simulink library "lib_SignalDiagnostic"  (R2017a)
settings: Solver=VariableStepAuto  StartTime=0.0  StopTime=10.0  RelTol=1e-3
libraries: simulink x35
settings Model: Creator=Di Russo  LastModifiedBy=Di Russo

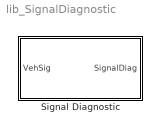
== system lib_SignalDiagnostic ==
  Signal Diagnostic : Subsystem

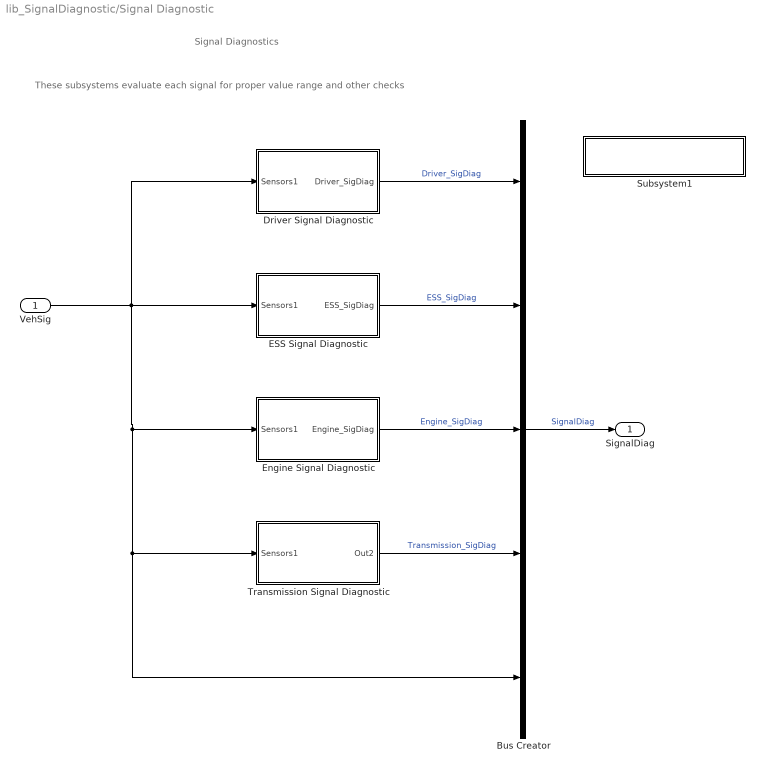
== system lib_SignalDiagnostic/Signal Diagnostic ==
  note: These subsystems evaluate each signal for proper value range and other checks
  note: Signal Diagnostics
  VehSig : Inport
  Bus Creator : BusCreator  Inputs=5
  Driver Signal Diagnostic : Subsystem
  ESS Signal Diagnostic : Subsystem
  Engine Signal Diagnostic : Subsystem
  Subsystem1 : Subsystem
      mask Display: fprintf('Signal Naming Rule')
  Transmission Signal Diagnostic : Subsystem
  SignalDiag : Outport
  wires:
  VehSig/1 -> ESS Signal Diagnostic/1(Sensors1), Driver Signal Diagnostic/1(Sensors1), Engine Signal Diagnostic/1(Sensors1), Bus Creator/5, Transmission Signal Diagnostic/1(Sensors1)
  Driver Signal Diagnostic/1(Driver_SigDiag) -> Bus Creator/1  "Driver_SigDiag"
  ESS Signal Diagnostic/1(ESS_SigDiag) -> Bus Creator/2  "ESS_SigDiag"
  Engine Signal Diagnostic/1(Engine_SigDiag) -> Bus Creator/3  "Engine_SigDiag"
  Transmission Signal Diagnostic/1(Out2) -> Bus Creator/4  "Transmission_SigDiag"
  Bus Creator/1 -> SignalDiag/1  "SignalDiag"

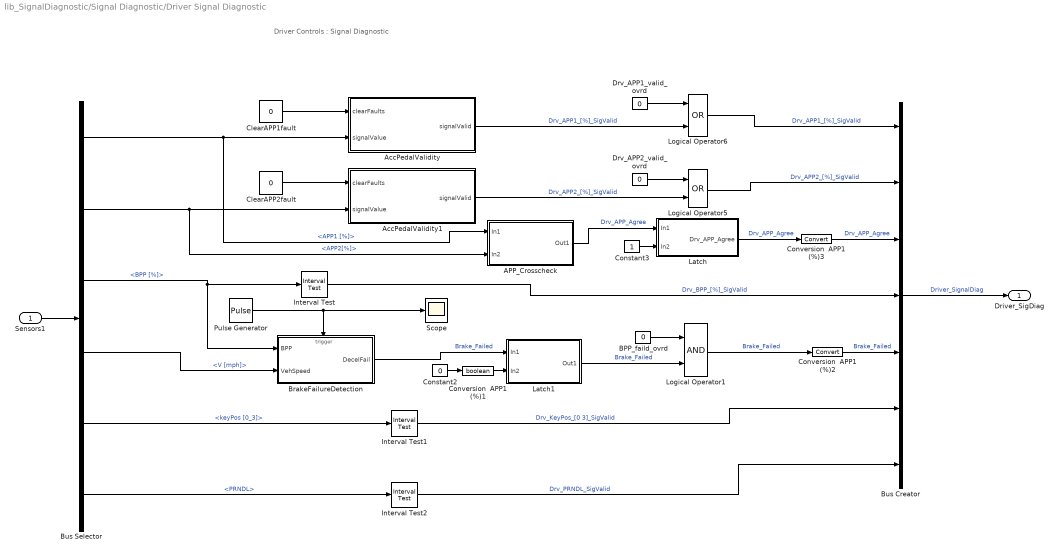
== system lib_SignalDiagnostic/Signal Diagnostic/Driver Signal Diagnostic ==
  note: Driver Controls : Signal Diagnostic
  Sensors1 : Inport
  APP_Crosscheck : Subsystem
  AccPedalValidity : Stateflow chart  TreatAsAtomicUnit=on
  AccPedalValidity1 : Stateflow chart  TreatAsAtomicUnit=on
  BPP_faild_ovrd : Constant  Value=0  OutDataTypeStr=boolean
  BrakeFailureDetection : Subsystem
  Bus Creator : BusCreator  Inputs=7
  Bus Selector : BusSelector  OutputSignals=DriverControls_Conv.APP1 [%],DriverControls_Conv.APP2[%],DriverControls_Conv.BPP [%],DriverControls_Conv.V [mph],DriverControls_Conv.keyPos [0_3],DriverControls_Conv.PRNDL
  ClearAPP1fault : Constant  Value=0
  ClearAPP2fault : Constant  Value=0
  Constant2 : Constant  Value=0
  Constant3 : Constant  OutDataTypeStr=boolean
  Conversion  APP1 (%)1 : DataTypeConversion  OutDataTypeStr=boolean
  Conversion  APP1 (%)2 : DataTypeConversion
  Conversion  APP1 (%)3 : DataTypeConversion
  Drv_APP1_valid_ovrd : Constant  Value=0  OutDataTypeStr=boolean
  Drv_APP2_valid_ovrd : Constant  Value=0  OutDataTypeStr=boolean
  Interval Test : simulink/Logic and Bit Operations/Interval Test  IntervalClosedRight=on  uplimit=100  IntervalClosedLeft=on  lowlimit=0  OutDataTypeStr=boolean
  Interval Test1 : simulink/Logic and Bit Operations/Interval Test  IntervalClosedRight=on  uplimit=3  IntervalClosedLeft=on  lowlimit=0  OutDataTypeStr=boolean
  Interval Test2 : simulink/Logic and Bit Operations/Interval Test  IntervalClosedRight=on  uplimit=4  IntervalClosedLeft=on  lowlimit=0  OutDataTypeStr=boolean
  Latch : Subsystem
  Latch1 : Subsystem
  Logical Operator1 : Logic  AllPortsSameDT=off  OutDataTypeStr=boolean
  Logical Operator5 : Logic  Operator=OR  AllPortsSameDT=off  OutDataTypeStr=boolean
  Logical Operator6 : Logic  Operator=OR  AllPortsSameDT=off  OutDataTypeStr=boolean
  Pulse Generator : DiscretePulseGenerator  PulseType=Time based  Period=0.1  PulseWidth=10
  Scope : Scope
  Driver_SigDiag : Outport
  wires:
  Sensors1/1 -> Bus Selector/1
  Bus Selector/1 -> AccPedalValidity/2(signalValue), APP_Crosscheck/1(In1)  "<APP1 [%]>"
  Bus Selector/2 -> AccPedalValidity1/2(signalValue), APP_Crosscheck/2(In2)  "<APP2[%]>"
  ClearAPP1fault/1 -> AccPedalValidity/1(clearFaults)
  ClearAPP2fault/1 -> AccPedalValidity1/1(clearFaults)
  Bus Selector/3 -> Interval Test/1, BrakeFailureDetection/1(BPP)  "<BPP [%]>"
  Bus Selector/5 -> Interval Test1/1  "<keyPos [0_3]>"
  Logical Operator6/1 -> Bus Creator/1  "Drv_APP1_[%]_SigValid"
  Interval Test/1 -> Bus Creator/4  "Drv_BPP_[%]_SigValid"
  Logical Operator5/1 -> Bus Creator/2  "Drv_APP2_[%]_SigValid"
  Bus Creator/1 -> Driver_SigDiag/1  "Driver_SignalDiag"
  Bus Selector/6 -> Interval Test2/1  "<PRNDL>"
  Constant3/1 -> Latch/2(In2)
  APP_Crosscheck/1(Out1) -> Latch/1(In1)  "Drv_APP_Agree"
  Bus Selector/4 -> BrakeFailureDetection/2(VehSpeed)  "<V [mph]>"
  Constant2/1 -> Conversion  APP1 (%)1/1
  Conversion  APP1 (%)1/1 -> Latch1/2(In2)
  BrakeFailureDetection/1(DecelFail) -> Latch1/1(In1)  "Brake_Failed"
  Interval Test2/1 -> Bus Creator/7  "Drv_PRNDL_SigValid"
  Drv_APP2_valid_ovrd/1 -> Logical Operator5/1
  AccPedalValidity1/1(signalValid) -> Logical Operator5/2  "Drv_APP2_[%]_SigValid"
  Drv_APP1_valid_ovrd/1 -> Logical Operator6/1
  AccPedalValidity/1(signalValid) -> Logical Operator6/2  "Drv_APP1_[%]_SigValid"
  Conversion  APP1 (%)3/1 -> Bus Creator/3  "Drv_APP_Agree"
  Conversion  APP1 (%)2/1 -> Bus Creator/5  "Brake_Failed"
  Interval Test1/1 -> Bus Creator/6  "Drv_KeyPos_[0 3]_SigValid"
  Latch/1(Drv_APP_Agree) -> Conversion  APP1 (%)3/1  "Drv_APP_Agree"
  Logical Operator1/1 -> Conversion  APP1 (%)2/1  "Brake_Failed"
  Latch1/1(Out1) -> Logical Operator1/2  "Brake_Failed"
  BPP_faild_ovrd/1 -> Logical Operator1/1
  Pulse Generator/1 -> BrakeFailureDetection/Trigger, Scope/1

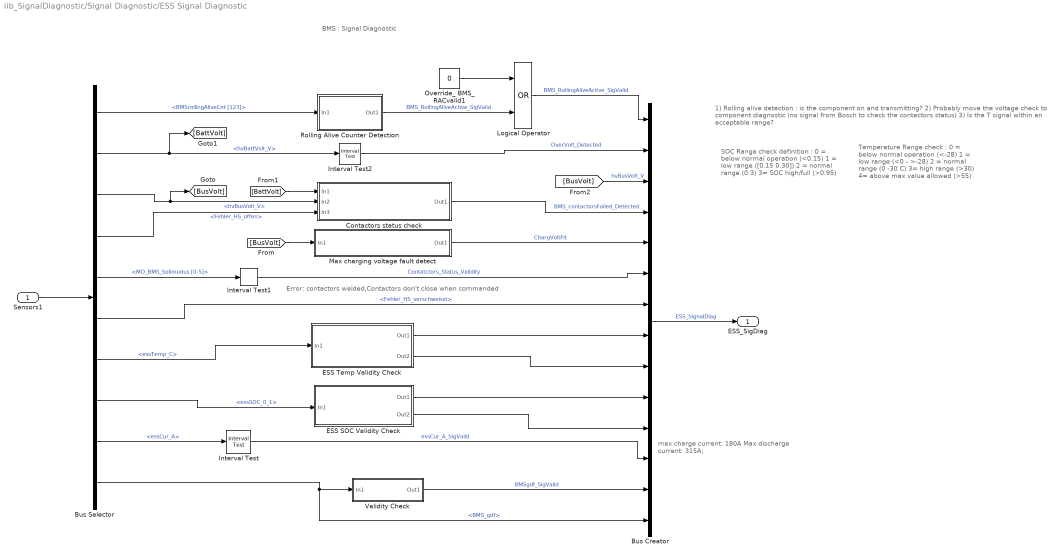
== system lib_SignalDiagnostic/Signal Diagnostic/ESS Signal Diagnostic ==
  note: max charge current: 180A
      | Max discharge current: 315A;
  note: Error: contactors welded,Contactors don't close when commanded
  note: Temperature Range check :
      | 0 = below normal operation (<-28)
      | 1 = low range (<0 - >-28)
      | 2 = normal range (0 -30 C)
      | 3= high range (>30)
      | 4= above max value allowed (>55)
  note: SOC Range check definition :
      | 0 = below normal operation (<0.15)
      | 1 = low range ([0.15 0.30])
      | 2 = normal range (0.3)
      | 3= SOC high/full (>0.95)
  note: 1) Rolling alive detection : is the component on and transmitting?
      | 2) Probably move the voltage check to component diagnostic (no signal from Bosch to check the contactors status)
      | 3) Is  the T signal within an acceptable range?
  note: BMS : Signal Diagnostic
  Sensors1 : Inport
  Bus Creator : BusCreator  Inputs=14
  Bus Selector : BusSelector  OutputSignals=BMS_Conv.BMSrollingAliveCnt [123],BMS_Conv.hvBattVolt_V,BMS_Conv.hvBusVolt_V,BMS_Conv.Fehler_HS_offen,BMS_Conv.MO_BMS_Sollmodus [0-5],BMS_Conv.Fehler_HS_verschweisst,BMS_Conv.essTemp_C,BMS_Conv.essSOC_0_1,BMS_Conv.essCur_A,BMS_Conv.BMS_gdf
  Contactors status check : Subsystem
  ESS SOC Validity Check : Subsystem
  ESS Temp Validity Check : Subsystem
  Interval Test : simulink/Logic and Bit Operations/Interval Test  IntervalClosedRight=on  uplimit=180  IntervalClosedLeft=on  lowlimit=-315  OutDataTypeStr=boolean
  Interval Test1 : simulink/Logic and Bit Operations/Interval Test  IntervalClosedRight=on  uplimit=7  IntervalClosedLeft=on  lowlimit=0  OutDataTypeStr=boolean
  Interval Test2 : simulink/Logic and Bit Operations/Interval Test  IntervalClosedRight=on  uplimit=430  IntervalClosedLeft=on  lowlimit=291  OutDataTypeStr=boolean
  Logical Operator : Logic  Operator=OR  AllPortsSameDT=off  OutDataTypeStr=boolean
  Max charging voltage fault detect : Subsystem
  Override_ BMS_RACvalid1 : Constant  Value=0
  Rolling Alive Counter Detection : Subsystem
  Validity Check : Subsystem
  ESS_SigDiag : Outport
  wires:
  Sensors1/1 -> Bus Selector/1
  Bus Selector/1 -> Rolling Alive Counter Detection/1(In1)  "<BMSrollingAliveCnt [123]>"
  Logical Operator/1 -> Bus Creator/1  "BMS_RollingAliveActive_SigValid"
  Bus Selector/2 -> Interval Test2/1, [BattVolt]  "<hvBattVolt_V>"
  Bus Creator/1 -> ESS_SigDiag/1  "ESS_SignalDiag"
  Bus Selector/9 -> Interval Test/1  "<essCur_A>"
  Interval Test/1 -> Bus Creator/12  "essCur_A_SigValid"
  Bus Selector/10 -> Bus Creator/14, Validity Check/1(In1)  "<BMS_gdf>"
  Validity Check/1(Out1) -> Bus Creator/13  "BMSgdf_SigValid"
  Bus Selector/8 -> ESS SOC Validity Check/1(In1)  "<essSOC_0_1>"
  ESS SOC Validity Check/1(Out1) -> Bus Creator/10
  ESS SOC Validity Check/2(Out2) -> Bus Creator/11
  Bus Selector/7 -> ESS Temp Validity Check/1(In1)  "<essTemp_C>"
  ESS Temp Validity Check/1(Out1) -> Bus Creator/8
  ESS Temp Validity Check/2(Out2) -> Bus Creator/9
  Bus Selector/3 -> Contactors status check/2(In2), [BusVolt]  "<hvBusVolt_V>"
  Bus Selector/4 -> Contactors status check/3(In3)  "<Fehler_HS_offen>"
  Contactors status check/1(Out1) -> Bus Creator/4  "BMS_contactorsFailed_Detected"
  Bus Selector/6 -> Bus Creator/7  "<Fehler_HS_verschweisst>"
  Bus Selector/5 -> Interval Test1/1  "<MO_BMS_Sollmodus [0-5]>"
  Interval Test1/1 -> Bus Creator/6  "Contatctors_Status_Validity"
  Interval Test2/1 -> Bus Creator/2  "OverVolt_Detected"
  [BattVolt] -> Contactors status check/1(In1)
  [BusVolt] -> Max charging voltage fault detect/1(In1)
  Max charging voltage fault detect/1(Out1) -> Bus Creator/5  "ChargVoltFlt"
  [BusVolt] -> Bus Creator/3  "hvBusVolt_V"
  Rolling Alive Counter Detection/1(Out1) -> Logical Operator/2  "BMS_RollingAliveActive_SigValid"
  Override_ BMS_RACvalid1/1 -> Logical Operator/1

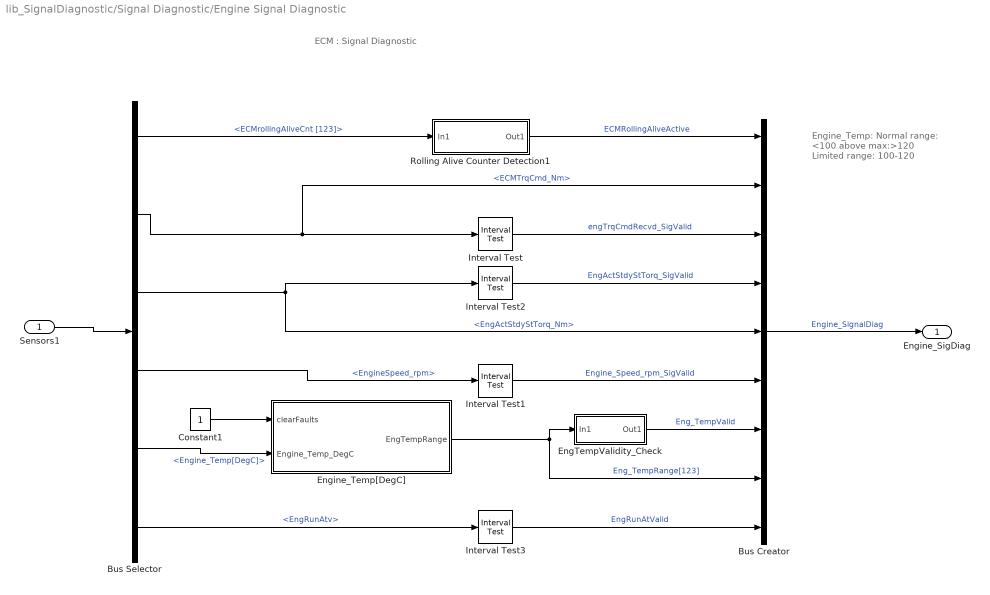
== system lib_SignalDiagnostic/Signal Diagnostic/Engine Signal Diagnostic ==
  note: ECM : Signal Diagnostic
  note: Engine_Temp:
      | Normal range: <100
      | above max:>120
      | Limited range: 100-120
  Sensors1 : Inport
  Bus Creator : BusCreator  Inputs=9
  Bus Selector : BusSelector  OutputSignals=ECM_Conv.ECMrollingAliveCnt [123],ECM_Conv.ECMTrqCmd_Nm,ECM_Conv.EngActStdyStTorq_Nm,ECM_Conv.EngineSpeed_rpm,ECM_Conv.Engine_Temp[DegC],ECM_Conv.EngRunAtv
  Constant1 : Constant
  EngTempValidity_Check : Subsystem
  Engine_Temp[DegC] : Stateflow chart  TreatAsAtomicUnit=on
  Interval Test : simulink/Logic and Bit Operations/Interval Test  IntervalClosedRight=on  uplimit=233  IntervalClosedLeft=on  lowlimit=0  OutDataTypeStr=boolean
  Interval Test1 : simulink/Logic and Bit Operations/Interval Test  IntervalClosedRight=on  uplimit=6500  IntervalClosedLeft=on  lowlimit=0  OutDataTypeStr=boolean
  Interval Test2 : simulink/Logic and Bit Operations/Interval Test  IntervalClosedRight=on  uplimit=233  IntervalClosedLeft=on  lowlimit=0  OutDataTypeStr=boolean
  Interval Test3 : simulink/Logic and Bit Operations/Interval Test  IntervalClosedRight=on  uplimit=1  IntervalClosedLeft=on  lowlimit=0  OutDataTypeStr=boolean
  Rolling Alive Counter Detection1 : Subsystem
  Engine_SigDiag : Outport
  wires:
  Sensors1/1 -> Bus Selector/1
  Bus Selector/1 -> Rolling Alive Counter Detection1/1(In1)  "<ECMrollingAliveCnt [123]>"
  Rolling Alive Counter Detection1/1(Out1) -> Bus Creator/1  "ECMRollingAliveActive"
  Bus Selector/2 -> Bus Creator/2, Interval Test/1  "<ECMTrqCmd_Nm>"
  Interval Test/1 -> Bus Creator/3  "engTrqCmdRecvd_SigValid"
  Bus Creator/1 -> Engine_SigDiag/1  "Engine_SignalDiag"
  Bus Selector/4 -> Interval Test1/1  "<EngineSpeed_rpm>"
  Interval Test1/1 -> Bus Creator/6  "Engine_Speed_rpm_SigValid"
  Bus Selector/3 -> Bus Creator/5, Interval Test2/1  "<EngActStdyStTorq_Nm>"
  Interval Test2/1 -> Bus Creator/4  "EngActStdyStTorq_SigValid"
  Bus Selector/5 -> Engine_Temp[DegC]/2(Engine_Temp_DegC)  "<Engine_Temp[DegC]>"
  Bus Selector/6 -> Interval Test3/1  "<EngRunAtv>"
  Interval Test3/1 -> Bus Creator/9  "EngRunAtValid"
  Constant1/1 -> Engine_Temp[DegC]/1(clearFaults)
  Engine_Temp[DegC]/1(EngTempRange) -> EngTempValidity_Check/1(In1), Bus Creator/8  "Eng_TempRange[123]"
  EngTempValidity_Check/1(Out1) -> Bus Creator/7  "Eng_TempValid"

== system lib_SignalDiagnostic/Signal Diagnostic/Subsystem1 ==
  note: Signal Valid Setting Rule
      | xxx_yyy_[z]_SigValid could be 0 or 1
      | 0: signal invalid
      | 1: signal vaild
  note: Signal Naming Rule
      | Example: xxx_yyy_[z]_SigValid
      | xxx: source of the signal (Drv, Clu, BCM, ECM, TCM, BMS and MCU)
      | yyy: description of the signal
      | z: unit of the signal (V, A, Nm, m/s, %, 01, 0123, etc.)

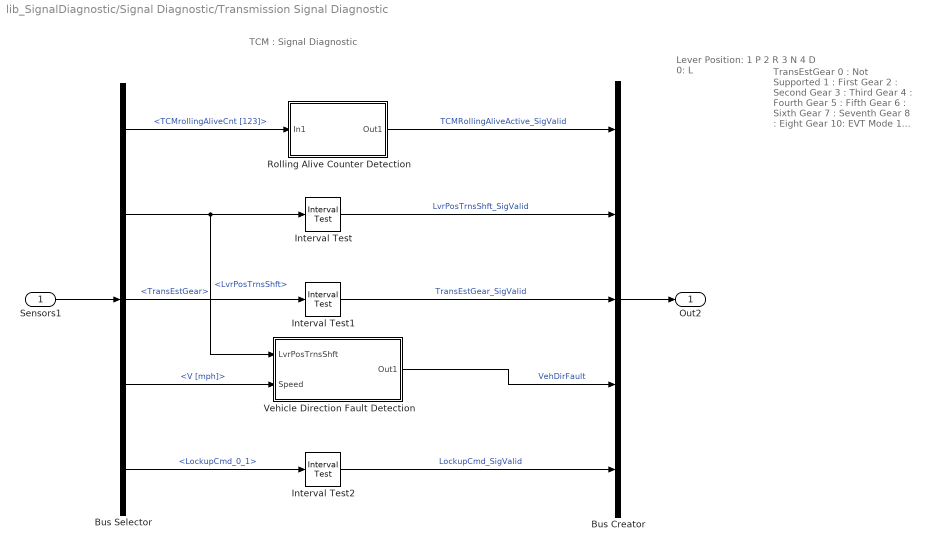
== system lib_SignalDiagnostic/Signal Diagnostic/Transmission Signal Diagnostic ==
  note: TCM : Signal Diagnostic
  note: TransEstGear
      | 0 : Not Supported
      | 1 : First Gear
      | 2 : Second Gear
      | 3 : Third Gear
      | 4 : Fourth Gear
      | 5 : Fifth Gear
      | 6 : Sixth Gear
      | 7 : Seventh Gear
      | 8 : Eight Gear
      | 10: EVT Mode 1
      | 11: EVT Mode 2
      | 12: CVT Forward Gear
      | 13: Neutral Gear
      | 14: Reverse Gear
      | 15: Park Gear
  note: Lever Position:
      | 1 P
      | 2 R
      | 3 N
      | 4 D
      | 0: L
  Sensors1 : Inport
  Bus Creator : BusCreator  Inputs=5
  Bus Selector : BusSelector  OutputSignals=TCM_Conv.TCMrollingAliveCnt [123],TCM_Conv.LvrPosTrnsShft,TCM_Conv.TransEstGear,DriverControls_Conv.V [mph],TCM_Conv.LockupCmd_0_1
  Interval Test : simulink/Logic and Bit Operations/Interval Test  IntervalClosedRight=on  uplimit=4  IntervalClosedLeft=on  lowlimit=0  OutDataTypeStr=boolean
  Interval Test1 : simulink/Logic and Bit Operations/Interval Test  IntervalClosedRight=on  uplimit=15  IntervalClosedLeft=on  lowlimit=0  OutDataTypeStr=boolean
  Interval Test2 : simulink/Logic and Bit Operations/Interval Test  IntervalClosedRight=on  uplimit=1  IntervalClosedLeft=on  lowlimit=0  OutDataTypeStr=boolean
  Rolling Alive Counter Detection : Subsystem
  Vehicle Direction Fault Detection : Subsystem
  Out2 : Outport
  wires:
  Bus Selector/4 -> Vehicle Direction Fault Detection/2(Speed)  "<V [mph]>"
  Sensors1/1 -> Bus Selector/1
  Bus Selector/1 -> Rolling Alive Counter Detection/1(In1)  "<TCMrollingAliveCnt [123]>"
  Rolling Alive Counter Detection/1(Out1) -> Bus Creator/1  "TCMRollingAliveActive_SigValid"
  Bus Creator/1 -> Out2/1
  Bus Selector/2 -> Vehicle Direction Fault Detection/1(LvrPosTrnsShft), Interval Test/1  "<LvrPosTrnsShft>"
  Bus Selector/3 -> Interval Test1/1  "<TransEstGear>"
  Bus Selector/5 -> Interval Test2/1  "<LockupCmd_0_1>"
  Interval Test/1 -> Bus Creator/2  "LvrPosTrnsShft_SigValid"
  Interval Test1/1 -> Bus Creator/3  "TransEstGear_SigValid"
  Interval Test2/1 -> Bus Creator/5  "LockupCmd_SigValid"
  Vehicle Direction Fault Detection/1(Out1) -> Bus Creator/4  "VehDirFault"

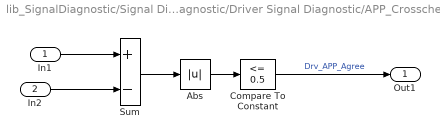
== system lib_SignalDiagnostic/Signal Diagnostic/Driver Signal Diagnostic/APP_Crosscheck ==
  In1 : Inport
  In2 : Inport  Port=2
  Abs : Abs
  Compare To Constant : simulink/Logic and Bit Operations/Compare To Constant  relop=<=  const=0.5  OutDataTypeStr=boolean
  Sum : Sum  Inputs=+-
  Out1 : Outport
  wires:
  Sum/1 -> Abs/1
  Abs/1 -> Compare To Constant/1
  In1/1 -> Sum/1
  In2/1 -> Sum/2
  Compare To Constant/1 -> Out1/1  "Drv_APP_Agree"

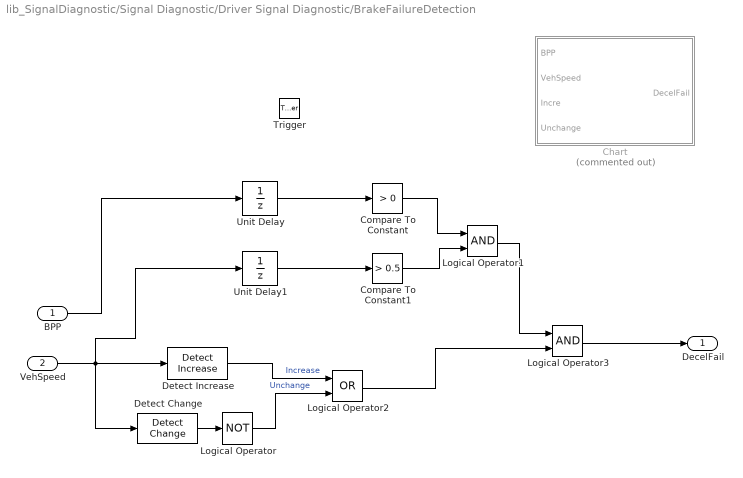
== system lib_SignalDiagnostic/Signal Diagnostic/Driver Signal Diagnostic/BrakeFailureDetection ==
  BPP : Inport
  VehSpeed : Inport  Port=2
  Trigger : TriggerPort  VariantControl=Variant  PortDimensions=1
  Chart : Stateflow chart  Commented=on  TreatAsAtomicUnit=on
  Compare To Constant : simulink/Logic and Bit Operations/Compare To Constant  relop=>  const=0  OutDataTypeStr=boolean
  Compare To Constant1 : simulink/Logic and Bit Operations/Compare To Constant  relop=>  const=0.5  OutDataTypeStr=boolean
  Detect Change : simulink/Logic and Bit Operations/Detect Change  vinit=0  InputProcessing=Inherited  OutDataTypeStr=boolean
  Detect Increase : simulink/Logic and Bit Operations/Detect Increase  vinit=0.0  InputProcessing=Inherited  OutDataTypeStr=boolean
  Logical Operator : Logic  Operator=NOT  AllPortsSameDT=off  OutDataTypeStr=boolean
  Logical Operator1 : Logic  AllPortsSameDT=off  OutDataTypeStr=boolean
  Logical Operator2 : Logic  Operator=OR  AllPortsSameDT=off  OutDataTypeStr=boolean
  Logical Operator3 : Logic  AllPortsSameDT=off  OutDataTypeStr=boolean
  Unit Delay : UnitDelay  SampleTime=-1
  Unit Delay1 : UnitDelay  SampleTime=-1
  DecelFail : Outport
  wires:
  VehSpeed/1 -> Unit Delay1/1, Detect Change/1, Detect Increase/1
  Detect Change/1 -> Logical Operator/1
  Compare To Constant/1 -> Logical Operator1/1
  Compare To Constant1/1 -> Logical Operator1/2
  BPP/1 -> Unit Delay/1
  Logical Operator1/1 -> Logical Operator3/1
  Detect Increase/1 -> Logical Operator2/1  "Increase"
  Logical Operator/1 -> Logical Operator2/2  "Unchange"
  Unit Delay/1 -> Compare To Constant/1
  Unit Delay1/1 -> Compare To Constant1/1
  Logical Operator2/1 -> Logical Operator3/2
  Logical Operator3/1 -> DecelFail/1

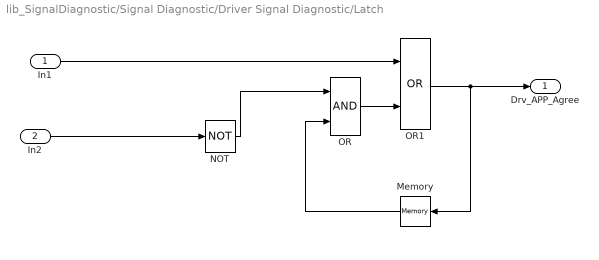
== system lib_SignalDiagnostic/Signal Diagnostic/Driver Signal Diagnostic/Latch ==
  In1 : Inport
  In2 : Inport  Port=2
  Memory : Memory
  NOT : Logic  Operator=NOT  OutDataTypeStr=boolean
  OR : Logic  OutDataTypeStr=boolean
  OR1 : Logic  Operator=OR  OutDataTypeStr=boolean
  Drv_APP_Agree : Outport
  wires:
  In1/1 -> OR1/1
  OR/1 -> OR1/2
  OR1/1 -> Drv_APP_Agree/1, Memory/1
  NOT/1 -> OR/1
  Memory/1 -> OR/2
  In2/1 -> NOT/1

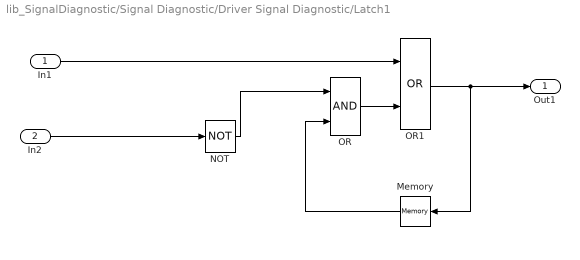
== system lib_SignalDiagnostic/Signal Diagnostic/Driver Signal Diagnostic/Latch1 ==
  In1 : Inport
  In2 : Inport  Port=2
  Memory : Memory
  NOT : Logic  Operator=NOT  OutDataTypeStr=boolean
  OR : Logic  OutDataTypeStr=boolean
  OR1 : Logic  Operator=OR  OutDataTypeStr=boolean
  Out1 : Outport
  wires:
  In2/1 -> NOT/1
  Memory/1 -> OR/2
  NOT/1 -> OR/1
  OR1/1 -> Memory/1, Out1/1
  OR/1 -> OR1/2
  In1/1 -> OR1/1

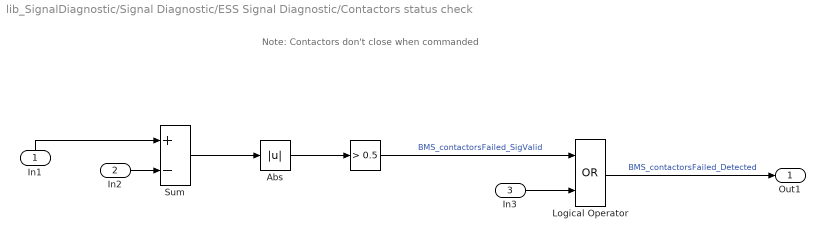
== system lib_SignalDiagnostic/Signal Diagnostic/ESS Signal Diagnostic/Contactors status check ==
  note: Note: Contactors don't close when commanded
  In1 : Inport
  In2 : Inport  Port=2
  In3 : Inport  Port=3
  " " : simulink/Logic and Bit Operations/Compare To Constant  relop=>  const=0.5  OutDataTypeStr=boolean
  Abs : Abs
  Logical Operator : Logic  Operator=OR  AllPortsSameDT=off  OutDataTypeStr=boolean
  Sum : Sum  Inputs=+-
  Out1 : Outport
  wires:
  " "/1 -> Logical Operator/1  "BMS_contactorsFailed_SigValid"
  In3/1 -> Logical Operator/2
  In2/1 -> Sum/2
  Abs/1 -> " "/1
  Sum/1 -> Abs/1
  Logical Operator/1 -> Out1/1  "BMS_contactorsFailed_Detected"
  In1/1 -> Sum/1

== system lib_SignalDiagnostic/Signal Diagnostic/ESS Signal Diagnostic/ESS SOC Validity Check ==
  In1 : Inport
  Constant1 : Constant
  essSOCValidity_Check : Subsystem
  essSOC_0_1Range : Stateflow chart  TreatAsAtomicUnit=on
  Out1 : Outport
  Out2 : Outport  Port=2
  wires:
  essSOCValidity_Check/1(Out1) -> Out1/1  "BMS_essSOC_0_1_SigValid"
  In1/1 -> essSOC_0_1Range/2(signalValue)
  Constant1/1 -> essSOC_0_1Range/1(clearFaults)
  essSOC_0_1Range/1(essSOCRange) -> Out2/1, essSOCValidity_Check/1(In1)

== system lib_SignalDiagnostic/Signal Diagnostic/ESS Signal Diagnostic/ESS Temp Validity Check ==
  In1 : Inport
  Constant : Constant
  essTsignalRange : Stateflow chart  TreatAsAtomicUnit=on
  essTsignalValidity_Check : Subsystem
  Out1 : Outport
  Out2 : Outport  Port=2
  wires:
  Constant/1 -> essTsignalRange/1(clearFaults)
  essTsignalValidity_Check/1(Out1) -> Out1/1  "BMS_essTemp_[degC]_SigValid"
  essTsignalRange/1(essTempRange) -> Out2/1, essTsignalValidity_Check/1(In1)  "essTempRange[0_4]"
  In1/1 -> essTsignalRange/2(signalValue)

== system lib_SignalDiagnostic/Signal Diagnostic/ESS Signal Diagnostic/Max charging voltage fault detect ==
  note: Note: When the ESS receives the energy from grid or regenerative braking,
      | the charging voltage to the inverter can not be bigger than 419V, otherwise the MCU will set to fault
  In1 : Inport
  " " : simulink/Logic and Bit Operations/Compare To Constant  relop=>  const=419  OutDataTypeStr=boolean
  Abs : Abs
  Compare To Zero : simulink/Logic and Bit Operations/Compare To Zero  relop=<  OutDataTypeStr=boolean
  Logical Operator : Logic  AllPortsSameDT=off  OutDataTypeStr=boolean
  Out1 : Outport
  wires:
  Compare To Zero/1 -> Logical Operator/2
  In1/1 -> Abs/1, Compare To Zero/1
  " "/1 -> Logical Operator/1
  Logical Operator/1 -> Out1/1
  Abs/1 -> " "/1

== system lib_SignalDiagnostic/Signal Diagnostic/ESS Signal Diagnostic/Rolling Alive Counter Detection ==
  In1 : Inport
  Chart : Stateflow chart  TreatAsAtomicUnit=on
  Constant : Constant  Value=0.01
  Constant1 : Constant  Value=0.01
  Detect Change : simulink/Logic and Bit Operations/Detect Change  vinit=1  InputProcessing=Inherited  OutDataTypeStr=boolean
  Out1 : Outport
  wires:
  Constant/1 -> Chart/2(CycleTime)
  Chart/1(flag) -> Out1/1
  Detect Change/1 -> Chart/1(PulseDetect)
  In1/1 -> Detect Change/1
  Constant1/1 -> Chart/3(tloop)

== system lib_SignalDiagnostic/Signal Diagnostic/ESS Signal Diagnostic/Validity Check ==
  In1 : Inport
  " Normal Operation" : simulink/Logic and Bit Operations/Compare To Constant  relop===  const=1  OutDataTypeStr=boolean
  Below Normal Operation : simulink/Logic and Bit Operations/Compare To Constant  relop===  const=0  OutDataTypeStr=boolean
  Logical Operator : Logic  Operator=OR  AllPortsSameDT=off  OutDataTypeStr=boolean
  Out1 : Outport
  wires:
  Logical Operator/1 -> Out1/1  "BMSgdf_SigValid"
  " Normal Operation"/1 -> Logical Operator/2
  Below Normal Operation/1 -> Logical Operator/1
  In1/1 -> " Normal Operation"/1, Below Normal Operation/1

== system lib_SignalDiagnostic/Signal Diagnostic/Engine Signal Diagnostic/EngTempValidity_Check ==
  In1 : Inport
  Above Normal Operation : simulink/Logic and Bit Operations/Compare To Constant  relop===  const=3  OutDataTypeStr=boolean
  Logical Operator1 : Logic  Operator=NOT  AllPortsSameDT=off  OutDataTypeStr=boolean
  Out1 : Outport
  wires:
  In1/1 -> Above Normal Operation/1
  Above Normal Operation/1 -> Logical Operator1/1
  Logical Operator1/1 -> Out1/1

== system lib_SignalDiagnostic/Signal Diagnostic/Engine Signal Diagnostic/Rolling Alive Counter Detection1 ==
  In1 : Inport
  Chart : Stateflow chart  TreatAsAtomicUnit=on
  Constant : Constant  Value=0.01
  Detect Change : simulink/Logic and Bit Operations/Detect Change  vinit=1  InputProcessing=Inherited  OutDataTypeStr=boolean
  Out1 : Outport
  wires:
  In1/1 -> Detect Change/1
  Detect Change/1 -> Chart/1(PulseDetect)
  Chart/1(flag) -> Out1/1
  Constant/1 -> Chart/2(CycleTime)

== system lib_SignalDiagnostic/Signal Diagnostic/Transmission Signal Diagnostic/Rolling Alive Counter Detection ==
  In1 : Inport
  Chart : Stateflow chart  TreatAsAtomicUnit=on
  Constant : Constant  Value=0.01
  Detect Change : simulink/Logic and Bit Operations/Detect Change  vinit=1  InputProcessing=Inherited  OutDataTypeStr=boolean
  Out1 : Outport
  wires:
  In1/1 -> Detect Change/1
  Detect Change/1 -> Chart/1(PulseDetect)
  Chart/1(flag) -> Out1/1
  Constant/1 -> Chart/2(CycleTime)

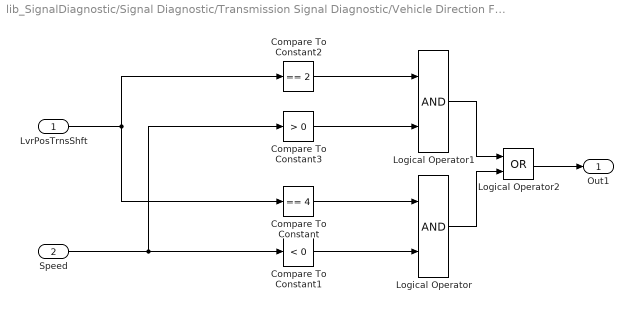
== system lib_SignalDiagnostic/Signal Diagnostic/Transmission Signal Diagnostic/Vehicle Direction Fault Detection ==
  LvrPosTrnsShft : Inport
  Speed : Inport  Port=2
  Compare To Constant : simulink/Logic and Bit Operations/Compare To Constant  relop===  const=4  OutDataTypeStr=boolean
  Compare To Constant1 : simulink/Logic and Bit Operations/Compare To Constant  relop=<  const=0  OutDataTypeStr=boolean
  Compare To Constant2 : simulink/Logic and Bit Operations/Compare To Constant  relop===  const=2  OutDataTypeStr=boolean
  Compare To Constant3 : simulink/Logic and Bit Operations/Compare To Constant  relop=>  const=0  OutDataTypeStr=boolean
  Logical Operator : Logic  AllPortsSameDT=off  OutDataTypeStr=boolean
  Logical Operator1 : Logic  AllPortsSameDT=off  OutDataTypeStr=boolean
  Logical Operator2 : Logic  Operator=OR  AllPortsSameDT=off  OutDataTypeStr=boolean
  Out1 : Outport
  wires:
  LvrPosTrnsShft/1 -> Compare To Constant2/1, Compare To Constant/1
  Speed/1 -> Compare To Constant3/1, Compare To Constant1/1
  Compare To Constant1/1 -> Logical Operator/2
  Compare To Constant/1 -> Logical Operator/1
  Compare To Constant2/1 -> Logical Operator1/1
  Compare To Constant3/1 -> Logical Operator1/2
  Logical Operator1/1 -> Logical Operator2/1
  Logical Operator/1 -> Logical Operator2/2
  Logical Operator2/1 -> Out1/1

== system lib_SignalDiagnostic/Signal Diagnostic/ESS Signal Diagnostic/ESS SOC Validity Check/essSOCValidity_Check ==
  In1 : Inport
  Above Normal Operation : simulink/Logic and Bit Operations/Compare To Constant  relop===  const=3  OutDataTypeStr=boolean
  Below Normal Operation : simulink/Logic and Bit Operations/Compare To Constant  relop===  const=0  OutDataTypeStr=boolean
  Logical Operator : Logic  Operator=OR  AllPortsSameDT=off  OutDataTypeStr=boolean
  Logical Operator1 : Logic  Operator=NOT  AllPortsSameDT=off  OutDataTypeStr=boolean
  Out1 : Outport
  wires:
  Logical Operator1/1 -> Out1/1
  Above Normal Operation/1 -> Logical Operator/2
  Below Normal Operation/1 -> Logical Operator/1
  Logical Operator/1 -> Logical Operator1/1
  In1/1 -> Below Normal Operation/1, Above Normal Operation/1

== system lib_SignalDiagnostic/Signal Diagnostic/ESS Signal Diagnostic/ESS Temp Validity Check/essTsignalValidity_Check ==
  In1 : Inport
  Above Normal Operation : simulink/Logic and Bit Operations/Compare To Constant  relop===  const=4  OutDataTypeStr=boolean
  Below Normal Operation : simulink/Logic and Bit Operations/Compare To Constant  relop===  const=0  OutDataTypeStr=boolean
  Logical Operator : Logic  Operator=OR  AllPortsSameDT=off  OutDataTypeStr=boolean
  Logical Operator1 : Logic  Operator=NOT  AllPortsSameDT=off  OutDataTypeStr=boolean
  Out1 : Outport
  wires:
  In1/1 -> Above Normal Operation/1, Below Normal Operation/1
  Logical Operator/1 -> Logical Operator1/1
  Below Normal Operation/1 -> Logical Operator/1
  Above Normal Operation/1 -> Logical Operator/2
  Logical Operator1/1 -> Out1/1

== stateflow chart lib_SignalDiagnostic/Signal Diagnostic/Driver Signal Diagnostic/AccPedalValidity ==
  state SignalHigh
    en: signalValid=0;
  state SignalInRange
  state SignalLow
    en:signalValid=0;
  SignalHigh -> SignalInRange : [signalValue<=100]
  SignalInRange -> SignalHigh [order 1] : [signalValue>102]
  SignalInRange -> SignalInRange [order 3] : [clearFaults==1]
      | {signalValid=1;}
  (default) -> SignalInRange : {signalValid=1;}
  SignalLow -> SignalInRange : [signalValue>0]
  SignalInRange -> SignalLow [order 2] : [signalValue<-0.5]
  data: clearFaults input; signalValue input; signalValid output

== stateflow chart lib_SignalDiagnostic/Signal Diagnostic/Driver Signal Diagnostic/AccPedalValidity1 ==
  state SignalHigh
    en: signalValid=0;
  state SignalInRange
  state SignalLow
    en:signalValid=0;
  SignalHigh -> SignalInRange : [signalValue<=100]
  SignalInRange -> SignalHigh [order 1] : [signalValue>102]
  SignalInRange -> SignalInRange [order 3] : [clearFaults==1]
      | {signalValid=1;}
  (default) -> SignalInRange : {signalValid=1;}
  SignalLow -> SignalInRange : [signalValue>0]
  SignalInRange -> SignalLow [order 2] : [signalValue<-0.5]
  data: clearFaults input; signalValue input; signalValid output

== stateflow chart lib_SignalDiagnostic/Signal Diagnostic/Driver Signal Diagnostic/BrakeFailureDetection/Chart ==
  state No_Fault
    en:
    DecelFail=0;
  state Detection_State
    en:
    Detection_state=1;
  state No_Fault1
    en:
    DecelFail=0;
  state Detection_State1
    en:
    Detection_state=2;
  state No_Fault2
    en:
    DecelFail=0;
  state Detection_State2
    en:
    Detection_state=3;
    du:
    DecelFail=1;
  (default) -> (junction 3)
  (junction 3) -> No_Fault [order 2]
  (junction 3) -> Detection_State [order 1] : [VehSpeed>0]
  Detection_State -> (junction 8)
  (junction 8) -> No_Fault1 [order 2]
  (junction 8) -> Detection_State1 [order 1] : [BPP>0]
  Detection_State1 -> (junction 15)
  (junction 15) -> No_Fault2 [order 2]
  (junction 15) -> Detection_State2 [order 1] : [Incre||Unchange]
  data: BPP input; VehSpeed input; Incre input; Unchange input; DecelFail output; Detection_state local

== stateflow chart lib_SignalDiagnostic/Signal Diagnostic/ESS Signal Diagnostic/ESS SOC Validity Check/essSOC_0_1Range ==
  state aboveMax
    en: essSOCRange=3;
  state NormalRange
    en: essSOCRange=2;
  state LowRange
    en:essSOCRange=1;
  state BelowNormal
    en: essSOCRange=0;
  aboveMax -> NormalRange : [signalValue<0.95]
  NormalRange -> aboveMax [order 1] : [signalValue>=0.95]
  NormalRange -> NormalRange [order 3] : [clearFaults==1]
      | {essSOCRange=2;}
  (default) -> NormalRange
  LowRange -> NormalRange [order 1] : [signalValue>0.3]
  NormalRange -> LowRange [order 2] : [signalValue<=0.3&&signalValue>0.15]
  LowRange -> BelowNormal [order 2] : [signalValue<=0.15]
  BelowNormal -> LowRange : [signalValue>0.15]
  data: clearFaults input; signalValue input; data local; essSOCRange output

== stateflow chart lib_SignalDiagnostic/Signal Diagnostic/ESS Signal Diagnostic/ESS Temp Validity Check/essTsignalRange ==
  state AboveMax
    en: essTempRange=4;
  state HighRange
    en: essTempRange=3;
  state NormalRange
    en: essTempRange=2;
  state LowRange
    en:essTempRange=1;
  state BelowNormal
    en: essTempRange=0;
  HighRange -> AboveMax [order 2] : [signalValue>55]
  AboveMax -> HighRange : [signalValue<55]
  HighRange -> NormalRange [order 1] : [signalValue<=30]
  NormalRange -> HighRange [order 1] : [signalValue>32]
  NormalRange -> NormalRange [order 3] : [clearFaults==1]
      | {essTempRange=2;}
  (default) -> NormalRange
  LowRange -> NormalRange [order 1] : [signalValue>=30]
  NormalRange -> LowRange [order 2] : [signalValue<0 ]
  LowRange -> BelowNormal [order 2] : [signalValue<-28]
  BelowNormal -> LowRange : [signalValue>28]
  data: clearFaults input; signalValue input; essTempRange output; data local

== stateflow chart lib_SignalDiagnostic/Signal Diagnostic/ESS Signal Diagnostic/Rolling Alive Counter Detection/Chart ==
  state Off
    en:flag=0;
  state Alive
    en:flag=1;
  state Dead
    en:flag=0;
  Alive -> Alive [order 1] : after(CycleTime-tloop,sec)
      | [PulseDetect==1]
  (default) -> Off
  Off -> Alive : [PulseDetect==1]
  Alive -> Dead [order 2] : after(CycleTime,sec)
  data: PulseDetect input; CycleTime input; flag output; tloop input

== stateflow chart lib_SignalDiagnostic/Signal Diagnostic/Engine Signal Diagnostic/Rolling Alive Counter Detection1/Chart ==
  state Off
    en:flag=0;
  state Alive
    en:flag=1;
  state Dead
    en:flag=0;
  Alive -> Alive [order 1] : after(CycleTime-tloop,sec)
      | [PulseDetect==1]
  (default) -> Off
  Off -> Alive : [PulseDetect==1]
  Alive -> Dead [order 2] : after(CycleTime,sec)
  data: PulseDetect input; CycleTime input; flag output; tloop parameter

== stateflow chart lib_SignalDiagnostic/Signal Diagnostic/Transmission Signal Diagnostic/Rolling Alive Counter Detection/Chart ==
  state Off
    en:flag=0;
  state Alive
    en:flag=1;
  state Dead
    en:flag=0;
  Alive -> Alive [order 1] : after(CycleTime-tloop,sec)
      | [PulseDetect==1]
  (default) -> Off
  Off -> Alive : [PulseDetect==1]
  Alive -> Dead [order 2] : after(CycleTime,sec)
  data: PulseDetect input; CycleTime input; flag output; tloop parameter

== stateflow chart lib_SignalDiagnostic/Signal Diagnostic/Engine Signal Diagnostic/Engine_Temp[DegC] ==
  state AboveMax
    en: EngTempRange=3;
  state HighRange
    en: EngTempRange=2;
  state NormalRange
    en: EngTempRange=1;
  HighRange -> AboveMax [order 2] : [Engine_Temp_DegC>120]
  AboveMax -> HighRange : [Engine_Temp_DegC<120]
  NormalRange -> HighRange [order 1] : [Engine_Temp_DegC>100&&Engine_Temp_DegC<120]
  HighRange -> NormalRange [order 1] : [Engine_Temp_DegC<=100]
  NormalRange -> NormalRange [order 2] : [clearFaults==1]
      | {EngTempRange=1;}
  (default) -> NormalRange
  data: clearFaults input; Engine_Temp_DegC input; EngTempRange output; data local
